simulink model "controller_electric"  (R2023b)
settings: Solver=VariableStepAuto  StartTime=0.0  StopTime=10.0  RelTol=1e-3
values from neighbouring files (symbols this model uses):
  ki = 20    [controller_el.m]    (also in controller_el_windup.m = 2117.9265; controllore_el2.m = 104; controllore_mag_lin.m = 2117.9265; validation_controller_freq.m = 2118)
  kp = 40    [controller_el.m]    (also in controller_el_windup.m = 46.0161; controllore_el2.m = 0.15; controllore_mag_lin.m = 46.0161; validation_controller_freq.m = 46)
  Lc = 0.3935    [Model_Parameter.m]    (also in Model_Parameter_version2.m = 0.3708; Stima_dei_parametri_Rc_Lc.m = mean(Lc_vect))
  Rtot = 9.089    [Model_Parameter.m]    (also in Model_Parameter_version2.m = 9.7585)
settings Model: Creator=lollo  LastModifiedBy=lollo

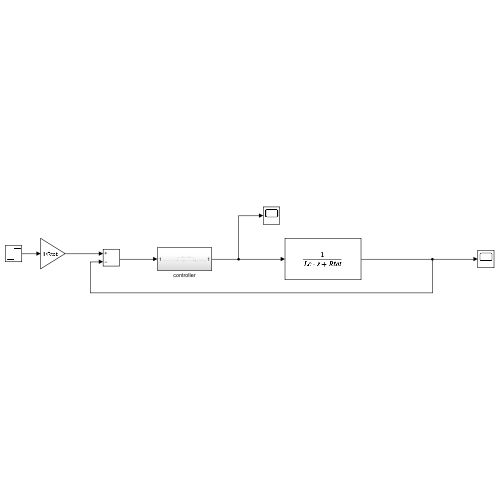
[thumbnail: Simulink's stored preview of the top-level diagram]
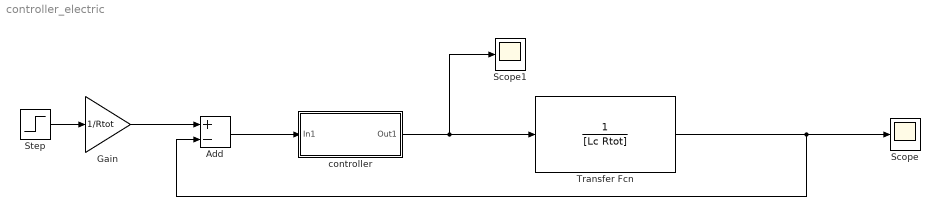
== system controller_electric ==
  Add : Sum  Inputs=+-
  Gain : Gain  Gain=1/Rtot
  Scope : Scope
  Scope1 : Scope
  Step : Step  Time=0  After=3  SampleTime=0
  Transfer Fcn : TransferFcn  Denominator=[Lc Rtot]
  controller : Subsystem
  wires:
  Transfer Fcn/1 -> Add/2, Scope/1
  controller/1(Out1) -> Scope1/1, Transfer Fcn/1
  Add/1 -> controller/1(In1)
  Step/1 -> Gain/1
  Gain/1 -> Add/1

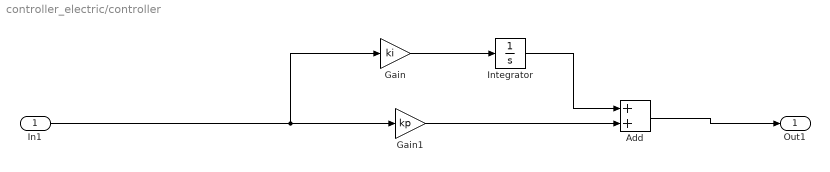
== system controller_electric/controller ==
  In1 : Inport
  Add : Sum
  Gain : Gain  Gain=ki
  Gain1 : Gain  Gain=kp
  Integrator : Integrator
  Out1 : Outport
  wires:
  Gain/1 -> Integrator/1
  Integrator/1 -> Add/1
  In1/1 -> Gain1/1, Gain/1
  Gain1/1 -> Add/2
  Add/1 -> Out1/1
